simulink model "base_model"  (R2020b)
settings: Solver=VariableStepAuto  StartTime=0.0  StopTime=30  RelTol=1e-3
values from neighbouring files (symbols this model uses):
  kd = 1.14032900506104    (= 1.14032900506)    [exp_tfest.m]
  ki = 0.134074922947779    (= 0.134074922948)    [exp_tfest.m]
  kn = 2.31488315878784    (= 2.31488315879)    [exp_tfest.m]
  kp = 1.0467641274631    (= 1.04676412746)    [exp_tfest.m]
libraries: pid_lib x1
settings Model: Creator=sprinkle  LastModifiedBy=fangyu
settings DebuggingCC: SFMachineParentedDataDiag=error

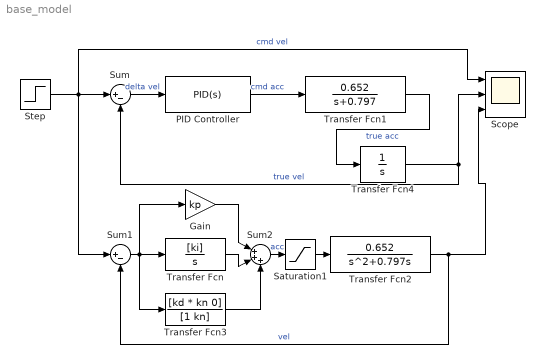
== system base_model ==
  Gain : Gain  Gain=kp
  PID Controller : pid_lib/PID Controller  Controller=PID  Form=Parallel  TimeDomain=Continuous-time  UseExternalTs=off  SampleTime=-1  IntegratorMethod=Forward Euler  FilterMethod=Forward Euler  ControllerParametersSource=internal  P=1.0467641274631  I=0.134074922947779  D=1.14032900506104  UseFilter=on  N=2.31488315878784  TunerSelectOption=Transfer Function Based (PID Tuner App)  InitialConditionSource=internal  InitialConditionForIntegrator=0  InitialConditionForFilter=0  DifferentiatorICPrevScaledInput=0  ExternalReset=none  TrackingMode=off  Kt=1  LimitOutput=on  SatLimitsSource=internal  UpperSaturationLimit=1.5  LowerSaturationLimit=-3  LinearizeAsGain=on  AntiWindupMode=clamping  Kb=1  POutMin=[]  POutMax=[]  IOutMin=[]  IOutMax=[]  DOutMin=[]  DOutMax=[]  NOutMin=[]  NOutMax=[]  SumOutMin=[]  SumOutMax=[]  SaturationOutMin=[]  SaturationOutMax=[]  PParamMin=[]  PParamMax=[]  IParamMin=[]  IParamMax=[]  DParamMin=[]  DParamMax=[]  NParamMin=[]  NParamMax=[]  KbParamMin=[]  KbParamMax=[]  KtParamMin=[]  KtParamMax=[]  KbOutMin=[]  KbOutMax=[]  KtOutMin=[]  KtOutMax=[]  IntegratorOutMin=[]  IntegratorOutMax=[]  FilterOutMin=[]  FilterOutMax=[]  SumI1OutMin=[]  SumI1OutMax=[]  SumI2OutMin=[]  SumI2OutMax=[]  SumI3OutMin=[]  SumI3OutMax=[]  SumI4OutMin=[]  SumI4OutMax=[]  SumDOutMin=[]  SumDOutMax=[]  DifferentiatorOutMin=[]  DifferentiatorOutMax=[]  FilterDiffOutCoefMin=[]  FilterDiffOutCoefMax=[]  ReciprocalOutMin=[]  ReciprocalOutMax=[]  SumDenOutMin=[]  SumDenOutMax=[]  SumNumOutMin=[]  SumNumOutMax=[]  DivideOutMin=[]  DivideOutMax=[]  UdiffTsProdOutMin=[]  UdiffTsProdOutMax=[]  NTsProdOutMin=[]  NTsProdOutMax=[]  UintegralTsProdOutMin=[]  UintegralTsProdOutMax=[]  UngainTsProdOutMin=[]  UngainTsProdOutMax=[]  IntegratorContinuousStateAttributes=''  IntegratorStateMustResolveToSignalObject=off  IntegratorRTWStateStorageClass=Auto  FilterContinuousStateAttributes=''  FilterStateMustResolveToSignalObject=off  FilterRTWStateStorageClass=Auto  ParallelPVariant=InternalParameters  IdealPVariant=Disabled  IVariant=InternalParameters  DVariant=InternalParameters  IntegratorVariant=Continuous  SatVariant=Enabled  AWVariant=ContClampingParallel  PCopyVariant=Disabled  TRVariant=Disabled  FdbkBlocksVariant=Forward  IdealPFdbkVariant=Disabled  SatFdbkVariant=Disabled  DerivativeFilterVariant=ContFilter  NVariant=InternalParameters  NCopyVariant=Disabled  FilterICVariant=InternalICsFilter  IntegratorICVariant=InternalICs  ExternalResetVariant=Disabled  TRSumVariant=Passthrough  SumFdbkVariant=Disabled  SumVariant=Sum_PID  TsampFilterVariant=InternalTs  TsampNgainVariant=Passthrough  TsampIntegralVariant=Passthrough  ExternalSaturationOutDataTypeStr=Inherit: Same as second input
  Saturation1 : Saturate  UpperLimit=1.5  LowerLimit=-3
  Scope : Scope  NumInputPorts=3
  Step : Step  SampleTime=0
  Sum : Sum  Inputs=|+-
  Sum1 : Sum  Inputs=|+-
  Sum2 : Sum  Inputs=|+++
  Transfer Fcn : TransferFcn  Numerator=[ki]  Denominator=[1 0]
  Transfer Fcn1 : TransferFcn  Numerator=[0.652]  Denominator=[1 0.797]
  Transfer Fcn2 : TransferFcn  Numerator=[0.652]  Denominator=[1 0.797 0]
  Transfer Fcn3 : TransferFcn  Numerator=[kd * kn 0]  Denominator=[1 kn]
  Transfer Fcn4 : TransferFcn  Denominator=[1 0]
  wires:
  Step/1 -> Sum1/1, Scope/1, Sum/1  "cmd vel"
  PID Controller/1 -> Transfer Fcn1/1  "cmd acc"
  Sum/1 -> PID Controller/1  "delta vel"
  Transfer Fcn2/1 -> Sum1/2, Scope/3  "vel"
  Sum1/1 -> Transfer Fcn3/1, Gain/1, Transfer Fcn/1
  Sum2/1 -> Saturation1/1  "acc"
  Transfer Fcn/1 -> Sum2/2
  Gain/1 -> Sum2/1
  Transfer Fcn3/1 -> Sum2/3
  Saturation1/1 -> Transfer Fcn2/1
  Transfer Fcn1/1 -> Transfer Fcn4/1  "true acc"
  Transfer Fcn4/1 -> Scope/2, Sum/2  "true vel"
